simulink model "proba"  (R2015b)
settings: Solver=VariableStepAuto  StartTime=0.0  StopTime=10.0  RelTol=1e-3
values from neighbouring files (symbols this model uses):
  A = [-100 0 0 ... (first row only)    [zad1.m]
  B = [1000 ... (first row only)    [zad1.m]
  C = [0 0 0.4]    [zad1.m]
  G = [-990720; 10957.5; -77.5]    [zad1.m]
settings Model: Creator=student  LastModifiedBy=student

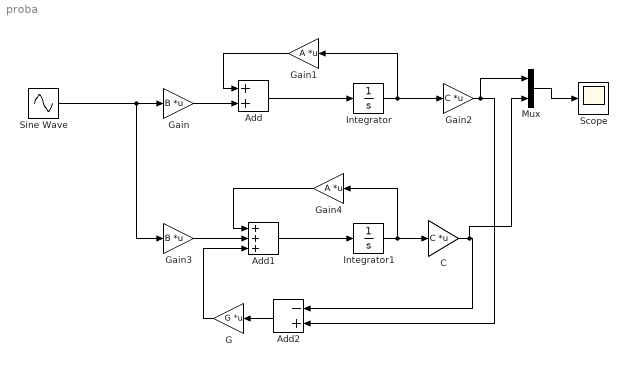
== system proba ==
  Add : Sum
  Add1 : Sum  Inputs=+++
  Add2 : Sum  Inputs=-+
  C : Gain  Gain=C  Multiplication=Matrix(K*u)
  G : Gain  Gain=G  Multiplication=Matrix(K*u)
  Gain : Gain  Gain=B  Multiplication=Matrix(K*u)
  Gain1 : Gain  Gain=A  Multiplication=Matrix(K*u)
  Gain2 : Gain  Gain=C  Multiplication=Matrix(K*u)
  Gain3 : Gain  Gain=B  Multiplication=Matrix(K*u)
  Gain4 : Gain  Gain=A  Multiplication=Matrix(K*u)
  Integrator : Integrator  InitialCondition=[0 0 0 ]
  Integrator1 : Integrator  InitialCondition=[1 1 1]
  Mux : Mux  Inputs=2
  Scope : Scope
  Sine Wave : Sin  SampleTime=0
  wires:
  Sine Wave/1 -> Gain3/1, Gain/1
  Add/1 -> Integrator/1
  Gain/1 -> Add/2
  Integrator/1 -> Gain2/1, Gain1/1
  Gain1/1 -> Add/1
  Gain2/1 -> Mux/1, Add2/2
  Gain3/1 -> Add1/2
  Add1/1 -> Integrator1/1
  Integrator1/1 -> C/1, Gain4/1
  Gain4/1 -> Add1/1
  C/1 -> Mux/2, Add2/1
  Add2/1 -> G/1
  G/1 -> Add1/3
  Mux/1 -> Scope/1
